simulink model "AirRefueling_Platform_ch10_4try"  (R2022a)
settings: Solver=ode3  StartTime=0.0  StopTime=300  FixedStep=0.01  RelTol=1e-5  AbsTol=1e-4  EnableMultiTasking=on
InitFcn:
  | F16_Init
values from neighbouring files (symbols this model uses):
  airSpeed = 393.72    [F16_Init.m]
  alpha0 = trimAlpha*180/pi    (= 6.62393794015)    [F16_Init.m]
  altitude = 9843    [F16_Init.m]
  b_ref = 30.0    (= 30)    [F16_Init.m]
  C = [ 1,0,0,zeros(1,15) ... (first row only)    [F16_Init.m]
  C2m = [C(1,:) ... (first row only)    [F16_Init.m]
  d_f_rc = [4.45;0;-3.81]    [F16_Init.m]
  d_pr_rc = [8.2;0.45;-3.3]    [F16_Init.m]
  dLEF = 0    [F16_Init.m]
  fi_flag = 1    [F16_Init.m]
  Kc = [ ... (first row only)    [F16_Init.m]
  Ki = zeros(4,3)    [F16_Init.m]
  Kp = zeros(4,18)    [F16_Init.m]
  mass = 636.94    [F16_Init.m]
  p0_pr = p0_rc + d_pr_rc    [F16_Init.m]
  p0_rc = [-28;0;0]    [F16_Init.m]
  trim_ail = 0.00874607850103852    (= 0.00874607850104)    [F16_Init.m]
  trim_control = [trim_thrust;trim_ele;trim_ail;trim_rud]    [F16_Init.m]
  trim_ele = -2.97973164860638    (= -2.97973164861)    [F16_Init.m]
  trim_rud = 0.0680302158182712    (= 0.0680302158183)    [F16_Init.m]
  trim_state1 = [trim_state;0;0;0;0;0;0]    [F16_Init.m]
  trim_thrust = 2279.08519954656    (= 2279.08519955)    [F16_Init.m]
  visual_err = [0;0;0]    [F16_Init.m]
undefined symbols (not defined in the file or in its folder): Cdr_, dockingPoint, dtheta10, dtheta20, F, height, k_reel, kd, l0, l1, l_density, Light, m0, Mdr, MIL, N, Rdr, Rl, STD, T_reel_initial, theta10, theta20, vt0
libraries: etargetslib x11, dspnetwork x10, aerolibconvert2 x6, aerolibasang x4, simulink x2, aerolibatmos2 x2, aerolibwind2 x2, aerolibobsolete x2, sharedtransform x2, aerolibutil x2, aerolibadyn x1, aerolibtransform2 x1
(part 3 of 3)

== matlab function AirRefueling_Platform_ch10_4try/Hose-drogue system/DRdynamics/Hose-Drogue1/MATLAB Function3 ==
  data: n input; alpha output; N parameter
function alpha = fcn(n, N)
% 计算两杆之间的弯折角度，用来粗略的验证恢复力的效果
alpha = zeros(1,N);
for i = 2:N
    mid = n(:,i-1)'*n(:,i);
    if abs(mid) > 1
        mid = mid/abs(mid);
    end
    alpha(i) = acos(mid)/pi*180;
end

== matlab function AirRefueling_Platform_ch10_4try/Receiver system/MATLAB Function ==
  settings: updateMethod=DISCRETE
  data: dd input; y output; dx input; t input; dockTime_out output
function [y, dockTime_out] = fcn(dd,dx,t)
%#codegen
%输入为xd，yd,-h
%调整为xd,h,yd

persistent aa;
if(isempty(aa))   %%aa(1:3)为锥套平衡位置,(4:6)为锥套实际位置或其滤波位置，(7:9)是锥管实际位置或其滤波位置；
    aa=zeros(9,1);
end

% 这个tt是用来对总体的时间逻辑进行控制的
persistent tt;
if(isempty(tt))
    tt=0;
end

persistent mm;    %%nn为前馈量
if(isempty(mm))
    mm=[0;0;0];
end

persistent nn;    %%nn为前馈量
if(isempty(nn))
    nn=[0;0;0];
end

persistent dockTime;
if(isempty(dockTime))
    dockTime = [0,0,0,0];
end

persistent dockCount;
if(isempty(dockCount))
    dockCount = 1;
end

t1=t-tt;
if t1<20
   y=[0;-2;6] ;
elseif t1<60
     y=[2;dx(2);dx(3)];  
     if t1>44&&t1<45
        aa(1:3)=y; 
     end
     if t1>58
         aa(1:3)=1/3*aa(1:3)+2/3*y;           %;做一个滤波，求出锥套的平衡点。
     end     
else
    
   deltaX=dd(1)-dx(1);
    if deltaX<-0.5 || deltaX>0
        nz=0;
        ny=0;
%     elseif deltaX<-0.5
%         nz=2*(deltaX+1);
%         ny=2*(deltaX+1);
    else
        nz=1;
        ny=1;
    end

    y=[dx(1)+nn(1);(1-ny)*(aa(2)+mm(2)+nn(2))+ny*(dx(2));(1-nz)*(aa(3)+mm(3)+nn(3))+nz*(dx(3))];
    %y=dx;
    
    
    if abs(dd(1)-dx(1))<0.01
       tt=t-21; 
       r=sqrt((dx(2)-dd(2))^2+(dx(3)-dd(3))^2);
       if r>0.2
           alpha=1/2;
       elseif r>0.1
           alpha=1/4;
       elseif r>0.05
           alpha=1/8;
       else
           alpha=0;
       end
       
       mm=(1-alpha)*mm+alpha*[0;(aa(5)-aa(2));(aa(6)-aa(3))];%+1/3*[0;(dx(2)-dd(2));-(dx(3)-dd(3))];
       nn=nn+0.5*[0;(aa(5)-aa(8));(aa(6)-aa(9))];
       if dockCount <= 4
           dockTime(dockCount) = t;
       end
       dockCount = dockCount + 1;
    elseif abs(dd(1)-dx(1))<0.4
        aa(4:6)=2/3*aa(4:6)+1/3*dx;
        aa(7:9)=2/3*aa(7:9)+1/3*dd;
    elseif abs(dd(1)-dx(1))<0.5
        aa(4:6)=dx;
        aa(7:9)=dd;
    end

end

dockTime_out = dockTime;

% 
% dx=[dx(1);dx(2);dx(3)];
% dd=[dd(1);dd(2);dd(3)];
% 
% t1=t-tt;
% % if t<5
% %     y=[2;-10;-4];
% % elseif t<10
% %     y=[1;10;4];
% % elseif t<20
% %     y=[4;-10;-4];
% if t1<20
%     y=[0;-6;-2];
% elseif t1<50
%      y=[4;dx(2);dx(3)];  
%      if t1>44&&t1<45
%         aa=y; 
%      end
%      if t1>45
%          aa=1/3*aa+2/3*y           %;做一个滤波，求出锥套的平衡点。
%      end
% else
%     y=[dx(1);aa(2)+mm(2);aa(3)+mm(3)];
%     %y=dx;
%     if abs(dd(1)-dx(1))<0.01
%        tt=t-21; 
%        mm=1/3*mm+2/3*[0;(aa(2)-dd(2));-(aa(3)-dd(3))]%+1/3*[0;(dx(2)-dd(2));-(dx(3)-dd(3))];
%     end
%         
% end

== matlab function AirRefueling_Platform_ch10_4try/Hose-drogue system/DRdynamics/Hose-Drogue1/Calculate the Acceleration of the Links1/MATLAB Function ==
  data: n input; m1 input; T output; m0 parameter; N parameter
function T = fcn(n,m1, m0,N)

% n = 连杆的方向向量，想上为正 向量3*N
% m = 连杆的质量 向量1*N

%%%%求张力t%%%%%%%%%%%%%%%%%%%%%%%%%%%%%%%%%%%%%%%%%%%%%%%%%%%%%%
T = zeros(N,N);

T(1,1) = 1;
T(1,2) = - n(:,1)'*n(:,2);
T(N,N-1) = -1/m0*n(:,N-1)'*n(:,N);
T(N,N) = 1/m0 + 1/m0;             %注意这里很重要！！

T(2,1) = -1/m1*n(:,1)'*n(:,2);
T(2,2) = 1/m1 + 1/m0;
T(2,3) = -1/m0*n(:,2)'*n(:,3);

for i = 3:N-1
    T(i,i-1) = -1/m0*n(:,i-1)'*n(:,i);
    T(i,i) = 1/m0 + 1/m0;
    T(i,i+1) = -1/m0*n(:,i)'*n(:,i+1);
end

== matlab function AirRefueling_Platform_ch10_4try/Tanker system/  ==
  data: u input; y output

function y = WindTurFromTank(u)
%#codegen

%横纵向气流角速度等下计算长度
c_lat=4;
c_lon=4;

%两端参考点
u1 = u+[0 ,c_lat ,0]';
u2 = u+[0 ,-c_lat, 0]';

yy1 = TankerVortexWindField(u1);
yy2 = TankerVortexWindField(u2);

%计算x轴向滚转角速度
yp = (yy1(3) - yy2(3))/4/c_lat;

u3=u+[c_lon, 0,0]';
u4=u+[-c_lon ,0,0]';
yy3 = TankerVortexWindField(u3);
yy4 = TankerVortexWindField(u4);

%俯仰角速度计算
yq = -(yy3(3) - yy4(3))/4/c_lon;

%偏航角速度设为0
yr = 0;

%质心处风场计算
y_uvw = TankerVortexWindField(u);


%y = [y_uvw(1);y_uvw(2);y_uvw(3);-yp;-yq;-yr]*0.5;
y = [y_uvw(1);y_uvw(2);y_uvw(3);-yp;-yq;-yr];

== matlab function AirRefueling_Platform_ch10_4try/Hose-drogue system/DRdynamics/HDU/MATLAB Function1 ==
  data: l1 input; l1initial input; dl1 input; flag1 output size=1; l1out output; dl1out output; ddl1 input; ddl1out output
function [flag1,l1out,dl1out,ddl1out] = fcn(l1,l1initial,dl1,ddl1)
% 如果第一根管子的长度比初始值大 或者 第一根管子的加速度>0 那么就是要控制了 flag从0变1开始积分
if (l1 > l1initial) || (l1 == l1initial && dl1 > 0)
    flag1 = 1;
    l1out = l1initial;
    dl1out = 0;
    ddl1out = 0;
else
    flag1 = 0;
    l1out = l1;
    dl1out = dl1;
    ddl1out = ddl1;
end

== matlab function AirRefueling_Platform_ch10_4try/Hose-drogue system/Bow Wave Effect/Bow Wave Effect Function ==
  data: x input; Fx output; y input; z input; Fy output; Fz output
function [Fx,Fy,Fz] = F_rc2dr(x,y,z)
Cx1 = 91.6170;
Cx2 = 0.3220;
Cx3 = 3.8870;
Cx4 = 2.7359;
Cx5 = 2.4939;
Cx6 = 309.7709;
Cx7 = 0.3237;
Cx8 = 0.3851;
Cx9 = 1.1471;

Cy1 = 223.3210;
Cy2 = 0.2082;
Cy3 = 0.8102;
Cy4 = 0.6555;

Cz1 = 173.2021;
Cz2 = 0.2141;
Cz3 = 0.5697;
Cz4 = 0.7038;

if x > 5.6493
    Fx = 0;
elseif x > 3.0893
    Fx = Cx1*(1-Cx2*(x-Cx3)^2)*exp(-y^2/Cx4)*exp(z/Cx5);
else
    Fx = Cx1*(1-Cx2*(x-Cx3)^2)*exp(-y^2/Cx4)*exp(z/Cx5)...
       + Cx6*(1-Cx7*x)*exp(-y^2/Cx8)*exp(z/Cx9);
end

if x > 4.8031
    Fy = 0;
else
    Fy = Cy1*(1-Cy2*x)*(y*exp(-y^2/Cy3))*exp(z/Cy4);
end

if x > 4.6275
    Fz = 0;
else
    Fz = -Cz1*(1-Cz2*x)*exp(-y^2/Cz3)*exp(z/Cz4);
end

== matlab function AirRefueling_Platform_ch10_4try/Hose-drogue system/Total Turbulence   ==
  data: u1 input; u input; y output
function y = Dr_wind2Frc(u1,u)
%#codegen

Ve=120;
rho = 0.98;
Q=0.5*rho*Ve^2;
S=0.38;
CD=0.81*0.8;

uu=u(1);
vv=u(2);
ww=u(3);

%beta = acos(sqrt(vv^2+ww^2)/abs(uu));
%theta = atan(ww/vv);

C_beta = 0.3979;

yx=rho*S*CD*Ve*uu;
yy=Q*S*C_beta*vv/Ve;
yz=Q*S*C_beta*ww/Ve;

% 这个y_v是有涡流+自然风所得到的速度换算成的位置偏移
y_v = [yx,yy,yz]';
y=[y_v;u1+y_v];

== matlab function AirRefueling_Platform_ch10_4try/Hose-drogue system/DRdynamics/HDU/MATLAB Function2 ==
  data: l_1 input; T0 input; Tt output size=1; t input; dl input; l1 parameter; k_reel parameter; kd parameter
function Tt = fcn(l_1,T0,t,dl, l1,k_reel,kd)
Treel = T0*(l_1/l1)^k_reel;
Tt = t - Treel - kd*dl;
